simulink model "three"  (R2014a)
settings: Solver=ode3  StartTime=0.0  StopTime=30  FixedStep=0.1  RelTol=1e-3
libraries: simulink x2
settings Model: Creator=Павел  LastModifiedBy=Павел
settings DataIOCC: InspectSignalLogs=on

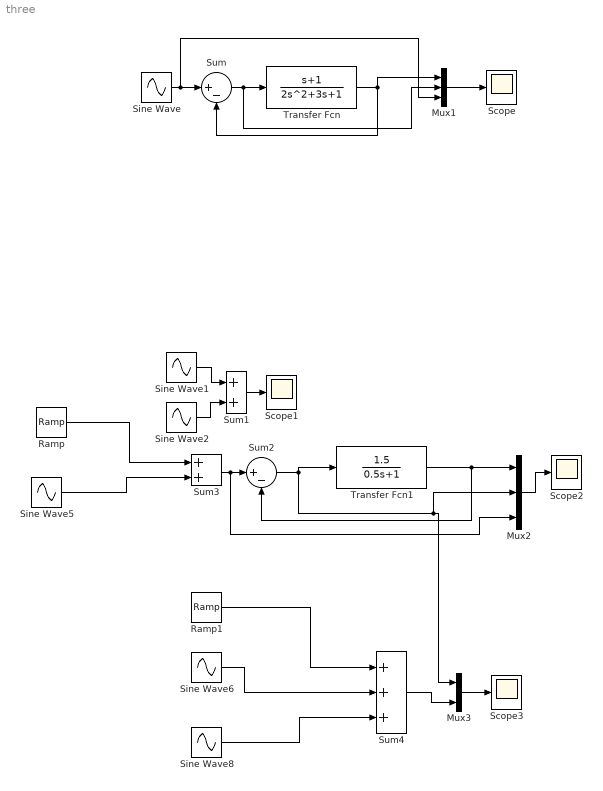
== system three ==
  Mux1 : Mux  Inputs=3
  Mux2 : Mux  Inputs=3
  Mux3 : Mux  Inputs=2
  Ramp : simulink/Sources/Ramp  slope=0.24  start=0  X0=0
  Ramp1 : simulink/Sources/Ramp  slope=0.2  start=0  X0=0
  Scope{,1..3} (4 alike) : Scope
      Scope settings: TimeRange=30
      Scope1 settings: TimeRange=30
      Scope2 settings: TimeRange=30  SaveName=ScopeData2
      Scope3 settings: TimeRange=100  YMin=0  YMax=20  SaveName=ScopeData3
  Sine Wave : Sin  Amplitude=0.6  Bias=3  Frequency=0.4  SampleTime=0
  Sine Wave1 : Sin  Amplitude=0.348  Bias=1.5  Frequency=0.4  SampleTime=0
  Sine Wave2 : Sin  Amplitude=0.12  Frequency=0.4  Phase=90  SampleTime=0
  Sine Wave5 : Sin  Amplitude=2  Frequency=0.1  Phase=90  SampleTime=0
  Sine Wave6 : Sin  Amplitude=0.024  Bias=0.06  Frequency=0.1  SampleTime=0
  Sine Wave8 : Sin  Amplitude=0.80048  Frequency=0.1  Phase=90  SampleTime=0
  Sum : Sum  Inputs=|+-
  Sum1 : Sum
  Sum2 : Sum  Inputs=|+-
  Sum3 : Sum
  Sum4 : Sum  Inputs=+++
  Transfer Fcn : TransferFcn  Numerator=[1 1]  Denominator=[2 3 1]
  Transfer Fcn1 : TransferFcn  Numerator=[1.5]  Denominator=[0.5 1]
  wires:
  Sum/1 -> Mux1/2, Transfer Fcn/1
  Transfer Fcn/1 -> Sum/2, Mux1/1
  Sine Wave1/1 -> Sum1/1
  Sine Wave2/1 -> Sum1/2
  Mux1/1 -> Scope/1
  Sine Wave/1 -> Mux1/3, Sum/1
  Mux2/1 -> Scope2/1
  Transfer Fcn1/1 -> Sum2/2, Mux2/1
  Sum3/1 -> Mux2/3, Sum2/1
  Sum2/1 -> Mux3/1, Mux2/2, Transfer Fcn1/1
  Ramp/1 -> Sum3/1
  Sine Wave5/1 -> Sum3/2
  Sum4/1 -> Mux3/2
  Sine Wave6/1 -> Sum4/2
  Sine Wave8/1 -> Sum4/3
  Ramp1/1 -> Sum4/1
  Sum1/1 -> Scope1/1
  Mux3/1 -> Scope3/1
